simulink model "nncontroller_5_50"  (R2021a)
(part 10 of 14)

  "IW{4,3}(50,:)'" : Constant  Value=[-0.95158718750855009194111744363908655941486358642578125;0.3782963226117204147413985992898233234882354736328125;0.400846694749627252551960054915980435907840728759765625;0.6730439046182377094140747431083582341670989990234375;-0.5651942366313758014939594431780278682708740234375;-0.21702293723794330304599498049356043338775634765625;-0.6994939862641833538958735516644082963466644287109375;-0.0816798824965896397287679064902476966381072998046875;-0.5719016828919747386095195906818844377994537353515625;-0.75251040908086519465314268018119037151336669921875;0.18930357643794337718645692802965641021728515625;-0.79585951449316194583616379532031714916229248046875;0.35117012879303499683913969420245848596096038818359375;-0.575745062984140520967457632650621235370635986328125;-0.595270142486898468092704206355847418308258056640625;0.0644897742469738854964589336304925382137298583984375;0.3349331447605423672797542167245410382747650146484375;0.9206779770980546562242352592875249683856964111328125;-0.1895882827554349336907080214587040245532989501953125;0.67050025300023519125858229017467238008975982666015625;0.1644488012169658952554840425364091061055660247802734375;-0.2421958042466481331178584923691232688724994659423828125;-0.90808065594589104652101241299533285200595855712890625;0.37539588933099621304023685297579504549503326416015625;-0.9536625824777196225312536626006476581096649169921875;0.55655750279535265434560642461292445659637451171875;0.143885692411657828415627591311931610107421875;-0.49627702975117149453154752336558885872364044189453125;0.350534505760690340281371391029097139835357666015625;-0.86696591045173232448206590561312623322010040283203125;0.743011185332303369932560599409043788909912109375;0.70867405317451648283366694158758036792278289794921875;0.9625546536904032723924728998099453747272491455078125;0.85082875624221798727120358307729475200176239013671875;-0.188963415959964908807933170464821159839630126953125;-0.035210371661677175580962284584529697895050048828125;-0.1027400611223512338909813479403965175151824951171875;0.30117104676955508413271900280960835516452789306640625;0.01009275895091803210146252922640996985137462615966796875;-0.1813370136564561307945808721342473290860652923583984375;-0.8958685760846913925803391975932754576206207275390625;0.0116029654669536075317637369153089821338653564453125;-0.62831409287320616474659118466661311686038970947265625;0.244165678119403539714227235890575684607028961181640625;-0.309955426261129485254741666722111403942108154296875;0.8321797883519728156187511558528058230876922607421875;0.8238776888166829959203596445149742066860198974609375;-0.54256266786282736358515421670745126903057098388671875;-0.222413662116213772801387449362664483487606048583984375;0.403156287700811410967816073025460354983806610107421875]
      mask Display: e = 0.06;c1 = [120 150 230]/255;c2 = ([120 150 230]+0)/383;c3 = ([120 150 230]+128)/383;patch([0 1 1 0],[0 0 1 1],c1);patch([0 1 1 1-e 1-e 0+e],[0 0 1 1-e 0+e 0+e],c2);patch([0 0 1 1-e 0+e 0+e],[0 1 1 1-e 1-e 0+e],c3);plot([0 1 1 0 0],[0 0 1 1 0]);disp('weights');
  "IW{4,3}(6,:)'" : Constant  Value=[0.78751746856938797947123021003790199756622314453125;-0.333235161357425813122290492174215614795684814453125;0.2026201601962955844982161579537205398082733154296875;-0.4684523397326805227436352652148343622684478759765625;-0.4250872143323809471127106007770635187625885009765625;-0.219578150481293032925123043241910636425018310546875;-0.4255570835394302253718024076079018414020538330078125;-0.458475300013506892327086461591534316539764404296875;-0.6872388102528272924018892808817327022552490234375;0.7555171386618890760900058012339286506175994873046875;0.2900404756725489807678286524605937302112579345703125;0.484909192138696376606077365067903883755207061767578125;0.7421621247430187917615285186911933124065399169921875;-0.0495746236903122916572783651645295321941375732421875;0.2327485650484817369942902587354183197021484375;0.7100475286185778944769708687090314924716949462890625;0.9842586819713392554120900967973284423351287841796875;-0.328126948659597683644051357987336814403533935546875;-0.88221413053549557758969967835582792758941650390625;0.406948172924789075555196404820890165865421295166015625;0.1505869152943757616203157567724701948463916778564453125;-0.00818606180615387424293061258140369318425655364990234375;-0.416990705819786089403322648649918846786022186279296875;-0.59133953190776533670458547931048087775707244873046875;-0.9291826152984097308973332474124617874622344970703125;-0.1947981515434170363132437842068611644208431243896484375;0.9912366054838599449539060515235178172588348388671875;-0.710504974254804633204685160308144986629486083984375;-0.4171211993744006196749296577763743698596954345703125;0.420579879262607203571633363026194274425506591796875;0.16267661019173385028580014477483928203582763671875;-0.86696055297430607566866456181742250919342041015625;-0.752385970311774787688818832975812256336212158203125;-0.94050819127969520483389942455687560141086578369140625;0.2984703641961090614387330788304097950458526611328125;0.051296281914861907580416300334036350250244140625;0.00082068813944413676608746754936873912811279296875;0.77897051385528126576929253133130259811878204345703125;0.30836368166160765813543775948346592485904693603515625;-0.1460313949979326064720908107119612395763397216796875;0.29801783925929548058064710858161561191082000732421875;0.7873445997398886841978082884452305734157562255859375;-0.65651592339721265290108931367285549640655517578125;0.28684920054759910357233820832334458827972412109375;0.89446636088867581548811358516104519367218017578125;-0.387433230241365389456831280767801217734813690185546875;0.55765722034091769199193322492646984755992889404296875;-0.0276736579807140246900498681270619272254407405853271484375;0.89322680703067536267525383664178662002086639404296875;0.74403188668467434840891883141011931002140045166015625]
      mask Display: e = 0.06;c1 = [120 150 230]/255;c2 = ([120 150 230]+0)/383;c3 = ([120 150 230]+128)/383;patch([0 1 1 0],[0 0 1 1],c1);patch([0 1 1 1-e 1-e 0+e],[0 0 1 1-e 0+e 0+e],c2);patch([0 0 1 1-e 0+e 0+e],[0 1 1 1-e 1-e 0+e],c3);plot([0 1 1 0 0],[0 0 1 1 0]);disp('weights');
  "IW{4,3}(7,:)'" : Constant  Value=[-0.4264681427911820588150249022874049842357635498046875;-0.858182072620006675123249806347303092479705810546875;-0.8340603604656544600715051274164579808712005615234375;0.4973565796534253902194677721126936376094818115234375;-0.7255106183500241723294266193988732993602752685546875;0.4810877643029678463193477000459097325801849365234375;0.5030552735275908293743896138039417564868927001953125;-0.3755592912510834491257583067636005580425262451171875;-0.811437958333129927268601022660732269287109375;0.2091062379235235635377421203884296119213104248046875;-0.5406996380607491659020524821244180202484130859375;-0.6545394493282972181447121329256333410739898681640625;0.23045786218899078079402897856198251247406005859375;0.1688915582862946518361013659159652888774871826171875;0.6012152243813273511108263846836052834987640380859375;-0.0108085759071017140087178631802089512348175048828125;0.062123006477989850537824167986400425434112548828125;-0.551336035061783302779758741962723433971405029296875;-0.8951355726501921683535556439892388880252838134765625;-0.896482938687404473654396497295238077640533447265625;0.3772351144452705806742187633062712848186492919921875;0.86116486107217493639609529054723680019378662109375;-0.4255069286566650621495000450522638857364654541015625;-0.170507032612538633742360616452060639858245849609375;0.2068767804119266973117419183836318552494049072265625;-0.108295492913722757322148027014918625354766845703125;0.412893343331278916963356095948256552219390869140625;0.4600896838446255632248949041240848600864410400390625;-0.174010165193382082549078404554165899753570556640625;-0.5825533110446752260713765281252562999725341796875;0.541310579280628534348807079368270933628082275390625;-0.6145033291533417152407992034568451344966888427734375;0.2968696445818235218894187710247933864593505859375;-0.934410924646730922660253781941719353199005126953125;0.5970868273202258880161252818652428686618804931640625;0.9842700072931018784316847813897766172885894775390625;-0.762739621688474311866912103141658008098602294921875;0.1927877868759220181260616300278343260288238525390625;0.3681983881897696875284964335151016712188720703125;-0.553499535841706968852804493508301675319671630859375;0.344652865473430214393602000200189650058746337890625;-0.35211250772713764689569870824925601482391357421875;-0.991304079940827254091573195182718336582183837890625;-0.750190879875885396899093393585644662380218505859375;-0.865838328649969124484186977497301995754241943359375;-0.5910433017973375502407407111604698002338409423828125;0.996601228575418662813945047673769295215606689453125;-0.961616331251665901191927332547493278980255126953125;0.5518880686856071360324449415202252566814422607421875;0.658846663777638230641287009348161518573760986328125]
      mask Display: e = 0.06;c1 = [120 150 230]/255;c2 = ([120 150 230]+0)/383;c3 = ([120 150 230]+128)/383;patch([0 1 1 0],[0 0 1 1],c1);patch([0 1 1 1-e 1-e 0+e],[0 0 1 1-e 0+e 0+e],c2);patch([0 0 1 1-e 0+e 0+e],[0 1 1 1-e 1-e 0+e],c3);plot([0 1 1 0 0],[0 0 1 1 0]);disp('weights');
  "IW{4,3}(8,:)'" : Constant  Value=[-0.65650212653692430198049123646342195570468902587890625;-0.2195810682015977288727981431293301284313201904296875;0.83947102459964140219739192616543732583522796630859375;0.4605039905349885831498113475390709936618804931640625;-0.9630439777879040708086222366546280682086944580078125;0.720335487849504740864858831628225743770599365234375;-0.8001927890614892735499097398133017122745513916015625;-0.60190292561296043771790209575556218624114990234375;0.4150538433636785651259515361743979156017303466796875;-0.4927628011742524183347313737613148987293243408203125;0.3499927702349860947350634887698106467723846435546875;-0.1891752363332557529407296215140377171337604522705078125;0.093908022347907404991929070092737674713134765625;0.5417495742319164975242529180832207202911376953125;-0.038636104586761366164182618376798927783966064453125;0.74698484734250480965300766911241225898265838623046875;-0.459354204369089080817190051675424911081790924072265625;0.65739285477904962906592345461831428110599517822265625;0.463375411868337583332078111197915859520435333251953125;0.043879381779363200999366512178312405012547969818115234375;-0.5052084550258639783493208597064949572086334228515625;0.6116850379363094614149076733156107366085052490234375;-0.59615901078961730519267803174443542957305908203125;-0.210742791759103875737224598196917213499546051025390625;-0.69449772725435654496806137103703804314136505126953125;-0.0189357103819347109829873687658619019202888011932373046875;-0.136417083212800438474232578300870954990386962890625;0.1203211202647417599198575999253080226480960845947265625;-0.0566110732885898304544980419450439512729644775390625;0.360668343526646617558384377844049595296382904052734375;0.49939713051086387363142193862586282193660736083984375;0.260143620258031227354678094343398697674274444580078125;0.848371925400467130629067469271831214427947998046875;-0.09370844596624601507972585068273474462330341339111328125;-0.0201513453607609083206853028968907892704010009765625;0.7224397528262496148698801334830932319164276123046875;-0.3745743263423142455081915613845922052860260009765625;-0.2989745826081742219315628972253762185573577880859375;0.11005105606762362324690940340587985701858997344970703125;0.98058752919594949215564838596037589013576507568359375;0.00918925634143625234828700598654904752038419246673583984375;-0.57315387956934404911635283497162163257598876953125;0.54783041317793335078789596082060597836971282958984375;0.42000397183685234114847162345540709793567657470703125;0.87229917890455144213746052628266625106334686279296875;-0.8796757285705039119960702009848318994045257568359375;-0.213945978616087606472007109914557076990604400634765625;-0.40763664316493031236632305081002414226531982421875;0.5969235809937980530293089032056741416454315185546875;-0.1176376192305655654646301400134689174592494964599609375]
      mask Display: e = 0.06;c1 = [120 150 230]/255;c2 = ([120 150 230]+0)/383;c3 = ([120 150 230]+128)/383;patch([0 1 1 0],[0 0 1 1],c1);patch([0 1 1 1-e 1-e 0+e],[0 0 1 1-e 0+e 0+e],c2);patch([0 0 1 1-e 0+e 0+e],[0 1 1 1-e 1-e 0+e],c3);plot([0 1 1 0 0],[0 0 1 1 0]);disp('weights');
  "IW{4,3}(9,:)'" : Constant  Value=[0.71220776746345204610832979597034864127635955810546875;-0.9838004782436848838500509373261593282222747802734375;-0.4060079031128565052455314798862673342227935791015625;0.852807580786446806087042205035686492919921875;0.90671488279771239593429754677345044910907745361328125;0.858652314476606282056536656455136835575103759765625;-0.9557094812840716269164431651006452739238739013671875;0.5360283523712576769781890106969512999057769775390625;0.530474255458407650820618073339574038982391357421875;0.5633304785467492248329790527350269258022308349609375;0.267779852910360549600454760366119444370269775390625;0.71779374858130273739931226373300887644290924072265625;-0.346073420523084152033987948016147129237651824951171875;0.435373483468067146162638891837559640407562255859375;0.6182877442450827043529670845600776374340057373046875;-0.090413630787127552412840714168851263821125030517578125;0.7530085479625849842477691709063947200775146484375;0.76348233733694093050559104085550643503665924072265625;-0.3027099109055757519826101997750811278820037841796875;0.53794208250024888595675065516843460500240325927734375;0.950123541759286371899406731245107948780059814453125;0.87725460785911024697014681805740110576152801513671875;-0.2187437265133535813088627719480427913367748260498046875;0.517435659062424946341707254759967327117919921875;-0.5689043150285530980880821516620926558971405029296875;0.431731902304381132129407205866300500929355621337890625;-0.777732917695507897093420979217626154422760009765625;-0.51350792746370010899426006290013901889324188232421875;-0.2059674290909878635602581198327243328094482421875;-0.1007567182827264484767937346987309865653514862060546875;-0.566470872220194987534114261507056653499603271484375;0.09208674012146535192702145877774455584585666656494140625;0.4572783919333585078703663384658284485340118408203125;-0.4900752762446798360684852013946510851383209228515625;0.54764893104469702933556618518196046352386474609375;-0.9173222729465504432511124832672066986560821533203125;0.068558947123779745425053988583385944366455078125;-0.006217831425509774169457788417503252276219427585601806640625;0.28779554762691550440223409168538637459278106689453125;0.3606964478557046493989446389605291187763214111328125;0.3638638195974392974818556467653252184391021728515625;-0.2913633750615740591882740773144178092479705810546875;-0.76627540137437766265549043964711017906665802001953125;0.471928240475669280584725129301659762859344482421875;-0.06807585352811797163585794123719097115099430084228515625;-0.690209618733953700342453885241411626338958740234375;0.7400203148090682692128439157386310398578643798828125;0.335129468205832059535254074944532476365566253662109375;-0.63672405329152603759013118178700096905231475830078125;-0.8405317519185120378466535839834250509738922119140625]
      mask Display: e = 0.06;c1 = [120 150 230]/255;c2 = ([120 150 230]+0)/383;c3 = ([120 150 230]+128)/383;patch([0 1 1 0],[0 0 1 1],c1);patch([0 1 1 1-e 1-e 0+e],[0 0 1 1-e 0+e 0+e],c2);patch([0 0 1 1-e 0+e 0+e],[0 1 1 1-e 1-e 0+e],c3);plot([0 1 1 0 0],[0 0 1 1 0]);disp('weights');
  Mux : Mux  Inputs=50
      mask Display: e = 0.06;c1 = [120 150 230]/255;c2 = ([120 150 230]+0)/383;c3 = ([120 150 230]+128)/383;patch([0 1 1 0],[0 0 1 1],c1);patch([0 1 1 1-e 1-e 0+e],[0 0 1 1-e 0+e 0+e],c2);patch([0 0 1 1-e 0+e 0+e],[0 1 1 1-e 1-e 0+e],c3);plot([0 1 1 0 0],[0 0 1 1 0]);disp('Mux');
  dotprod{1..50} (50 alike) : neural/Weight Functions/dotprod
  "lz{4,3}" : Outport
      mask Display: e = 0.06;c1 = [120 230 180]/255;c2 = ([120 230 180]+0)/(256+128);c3 = ([120 230 180]+128)/(256+128);patch([0 1 1 0],[0 0 1 1],c1);patch([0 1 1 1-e 1-e 0+e],[0 0 1 1-e 0+e 0+e],c2);patch([0 0 1 1-e 0+e 0+e],[0 1 1 1-e 1-e 0+e],c3);plot([0 1 1 0 0],[0 0 1 1 0]);
  wires:
  "IW{4,3}(1,:)'"/1 -> dotprod1/1
  "ad{4,3}"/1 -> dotprod1/2, dotprod2/2, dotprod3/2, dotprod4/2, dotprod5/2, dotprod6/2, dotprod7/2, dotprod8/2, dotprod9/2, dotprod10/2, dotprod11/2, dotprod12/2, dotprod13/2, dotprod14/2, dotprod15/2, dotprod16/2, dotprod17/2, dotprod18/2, dotprod19/2, dotprod20/2, dotprod21/2, dotprod22/2, dotprod23/2, dotprod24/2, dotprod25/2, dotprod26/2, dotprod27/2, dotprod28/2, dotprod29/2, dotprod30/2, dotprod31/2, dotprod32/2, dotprod33/2, dotprod34/2, dotprod35/2, dotprod36/2, dotprod37/2, dotprod38/2, dotprod39/2, dotprod40/2, dotprod41/2, dotprod42/2, dotprod43/2, dotprod44/2, dotprod45/2, dotprod46/2, dotprod47/2, dotprod48/2, dotprod49/2, dotprod50/2
  dotprod1/1 -> Mux/1
  "IW{4,3}(2,:)'"/1 -> dotprod2/1
  dotprod2/1 -> Mux/2
  "IW{4,3}(3,:)'"/1 -> dotprod3/1
  dotprod3/1 -> Mux/3
  "IW{4,3}(4,:)'"/1 -> dotprod4/1
  dotprod4/1 -> Mux/4
  "IW{4,3}(5,:)'"/1 -> dotprod5/1
  dotprod5/1 -> Mux/5
  "IW{4,3}(6,:)'"/1 -> dotprod6/1
  dotprod6/1 -> Mux/6
  "IW{4,3}(7,:)'"/1 -> dotprod7/1
  dotprod7/1 -> Mux/7
  "IW{4,3}(8,:)'"/1 -> dotprod8/1
  dotprod8/1 -> Mux/8
  "IW{4,3}(9,:)'"/1 -> dotprod9/1
  dotprod9/1 -> Mux/9
  "IW{4,3}(10,:)'"/1 -> dotprod10/1
  dotprod10/1 -> Mux/10
  "IW{4,3}(11,:)'"/1 -> dotprod11/1
  dotprod11/1 -> Mux/11
  "IW{4,3}(12,:)'"/1 -> dotprod12/1
  dotprod12/1 -> Mux/12
  "IW{4,3}(13,:)'"/1 -> dotprod13/1
  dotprod13/1 -> Mux/13
  "IW{4,3}(14,:)'"/1 -> dotprod14/1
  dotprod14/1 -> Mux/14
  "IW{4,3}(15,:)'"/1 -> dotprod15/1
  dotprod15/1 -> Mux/15
  "IW{4,3}(16,:)'"/1 -> dotprod16/1
  dotprod16/1 -> Mux/16
  "IW{4,3}(17,:)'"/1 -> dotprod17/1
  dotprod17/1 -> Mux/17
  "IW{4,3}(18,:)'"/1 -> dotprod18/1
  dotprod18/1 -> Mux/18
  "IW{4,3}(19,:)'"/1 -> dotprod19/1
  dotprod19/1 -> Mux/19
  "IW{4,3}(20,:)'"/1 -> dotprod20/1
  dotprod20/1 -> Mux/20
  "IW{4,3}(21,:)'"/1 -> dotprod21/1
  dotprod21/1 -> Mux/21
  "IW{4,3}(22,:)'"/1 -> dotprod22/1
  dotprod22/1 -> Mux/22
  "IW{4,3}(23,:)'"/1 -> dotprod23/1
  dotprod23/1 -> Mux/23
  "IW{4,3}(24,:)'"/1 -> dotprod24/1
  dotprod24/1 -> Mux/24
  "IW{4,3}(25,:)'"/1 -> dotprod25/1
  dotprod25/1 -> Mux/25
  "IW{4,3}(26,:)'"/1 -> dotprod26/1
  dotprod26/1 -> Mux/26
  "IW{4,3}(27,:)'"/1 -> dotprod27/1
  dotprod27/1 -> Mux/27
  "IW{4,3}(28,:)'"/1 -> dotprod28/1
  dotprod28/1 -> Mux/28
  "IW{4,3}(29,:)'"/1 -> dotprod29/1
  dotprod29/1 -> Mux/29
  "IW{4,3}(30,:)'"/1 -> dotprod30/1
  dotprod30/1 -> Mux/30
  "IW{4,3}(31,:)'"/1 -> dotprod31/1
  dotprod31/1 -> Mux/31
  "IW{4,3}(32,:)'"/1 -> dotprod32/1
  dotprod32/1 -> Mux/32
  "IW{4,3}(33,:)'"/1 -> dotprod33/1
  dotprod33/1 -> Mux/33
  "IW{4,3}(34,:)'"/1 -> dotprod34/1
  dotprod34/1 -> Mux/34
  "IW{4,3}(35,:)'"/1 -> dotprod35/1
  dotprod35/1 -> Mux/35
  "IW{4,3}(36,:)'"/1 -> dotprod36/1
  dotprod36/1 -> Mux/36
  "IW{4,3}(37,:)'"/1 -> dotprod37/1
  dotprod37/1 -> Mux/37
  "IW{4,3}(38,:)'"/1 -> dotprod38/1
  dotprod38/1 -> Mux/38
  "IW{4,3}(39,:)'"/1 -> dotprod39/1
  dotprod39/1 -> Mux/39
  "IW{4,3}(40,:)'"/1 -> dotprod40/1
  dotprod40/1 -> Mux/40
  "IW{4,3}(41,:)'"/1 -> dotprod41/1
  dotprod41/1 -> Mux/41
  "IW{4,3}(42,:)'"/1 -> dotprod42/1
  dotprod42/1 -> Mux/42
  "IW{4,3}(43,:)'"/1 -> dotprod43/1
  dotprod43/1 -> Mux/43
  "IW{4,3}(44,:)'"/1 -> dotprod44/1
  dotprod44/1 -> Mux/44
  "IW{4,3}(45,:)'"/1 -> dotprod45/1
  dotprod45/1 -> Mux/45
  "IW{4,3}(46,:)'"/1 -> dotprod46/1
  dotprod46/1 -> Mux/46
  "IW{4,3}(47,:)'"/1 -> dotprod47/1
  dotprod47/1 -> Mux/47
  "IW{4,3}(48,:)'"/1 -> dotprod48/1
  dotprod48/1 -> Mux/48
  "IW{4,3}(49,:)'"/1 -> dotprod49/1
  dotprod49/1 -> Mux/49
  "IW{4,3}(50,:)'"/1 -> dotprod50/1
  dotprod50/1 -> Mux/50
  Mux/1 -> "lz{4,3}"/1
